simulink model "neuron_plots"  (R2022a)
settings: Solver=VariableStepAuto  StartTime=0.0  StopTime=10  RelTol=1e-3
libraries: neuromorphic_blocks x2
settings Model: Creator=chris  LastModifiedBy=chris

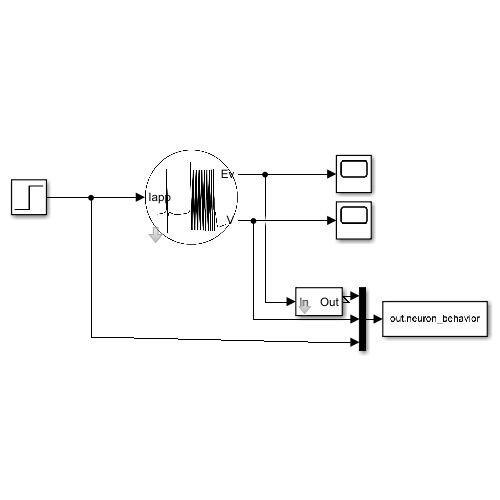
[thumbnail: Simulink's stored preview of the top-level diagram]
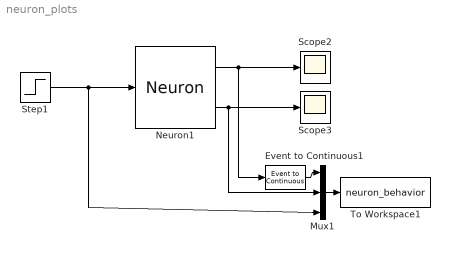
== system neuron_plots ==
  Event to Continuous1 : neuromorphic_blocks/Events Transmission Blocks/Event to Continuous  gain=1
      settings: SourceProductName=Neuromorphic Toolbox
  Mux1 : Mux  Inputs=3
  Neuron1 : neuromorphic_blocks/Neural Blocks/Neuron  gfm_source=Internal  gfm=3  gsp_source=Internal  gsp=6  gsm_source=Internal  gsm=2  gup_source=Internal  gup=5  gum_source=Internal  gum=2  dfm=0  dsp=0.5  dsm=-0.5  dup=-0.5  dum=-1  mfm=1  msp=1  msm=1  mup=1  mum=1  timescale=0.004  rel_membrane=0.1  rel_fast=0.1  rel_slow=4  rel_ultraslow=200  Iapp_base=-0.2  V0=-1.2  tresh=0  output=Both
      settings: SourceProductName=Neuromorphic Toolbox
  Scope2 : Scope
  Scope3 : Scope
  Step1 : Step  Time=5  After=0.02  SampleTime=0
  To Workspace1 : ToWorkspace  VariableName=neuron_behavior  SaveFormat=Structure With Time  SampleTime=-1
  wires:
  Event to Continuous1/1 -> Mux1/1
  Mux1/1 -> To Workspace1/1
  Neuron1/1 -> Event to Continuous1/1, Scope2/1
  Step1/1 -> Mux1/3, Neuron1/1
  Neuron1/2 -> Scope3/1, Mux1/2
